simulink model "MIXER"  (R2017a)
settings: Solver=VariableStepAuto  StartTime=0.0  StopTime=50.0  RelTol=1e-3
values from neighbouring files (symbols this model uses):
  a = 1.8    [Integral.m]    (also in Koshi.m = 0; MNK.m = -5; Spline_1_0.m = -5; Spline_2_1.m = -5)
  c1 = 1    [data_mixer.m]    (also in data_mixer_for_gui.m)
  c2 = 2    [data_mixer.m]    (also in data_mixer_for_gui.m; my.m = 0.4)
  cz = 1.25    [data_mixer.m]
  F1z = uz(1)    [data_mixer.m]    (also in data_mixer_for_gui.m)
  F2z = uz(2)    [data_mixer.m]    (also in data_mixer_for_gui.m)
  Fz = 0.02    [data_mixer.m]
  k = k + 1    (= 2)    [complex_ikf.m]    (also in data_mixer.m = 0.02; data_mixer_for_gui.m = 0.02; my.m = 5)
  k1 = -10    [data_mixer.m]
  k2 = -10    [data_mixer.m]
  S = @(k)(((b1-a).^(k+1-betta))-((b1-b).^(k+1-betta)))./(k+1-betta)    [Gauss.m]    (also in Integral.m = @(k)((1/2).^(k+2/5))./(k+2/5); Nuton_Kotes.m; data_mixer.m = 1; data_mixer_for_gui.m = 1)
  X_ini = [1.5 0.5].'    [data_mixer.m]
undefined symbols (not defined in the file or in its folder): F_for_MIXER
settings Model: Creator=User  LastModifiedBy=User

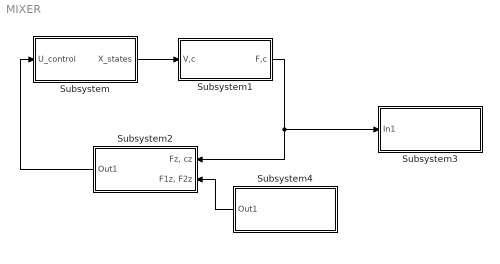
== system MIXER ==
  Subsystem : Subsystem
      mask Display:
      | color('blue');
      | disp('MIXER');
  Subsystem1 : Subsystem
      mask Display:
      | color('red');
      | disp('MEARSUREMENTS');
  Subsystem2 : Subsystem
      mask Display:
      | color('blue');
      | disp('CONTROL');
  Subsystem3 : Subsystem
      mask Display:
      | color('blue');
      | disp('DISPLAY');
  Subsystem4 : Subsystem
      mask Display:
      | color('blue');
      | disp('COMMAND\nSIGNAL');
  wires:
  Subsystem/1(X_states) -> Subsystem1/1(V,c)
  Subsystem1/1(F,c) -> Subsystem3/1(In1), Subsystem2/1("Fz, cz")
  Subsystem2/1(Out1) -> Subsystem/1(U_control)
  Subsystem4/1(Out1) -> Subsystem2/2("F1z, F2z")

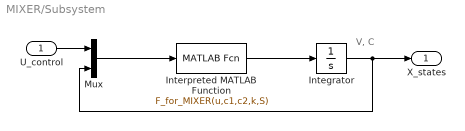
== system MIXER/Subsystem ==
  note: V, C
  U_control : Inport
  Integrator : Integrator  InitialCondition=X_ini
  Interpreted MATLAB Function : MATLABFcn  MATLABFcn=F_for_MIXER(u,c1,c2,k,S)
  Mux : Mux  Inputs=2
  X_states : Outport
  wires:
  Interpreted MATLAB Function/1 -> Integrator/1
  Integrator/1 -> Mux/2, X_states/1
  U_control/1 -> Mux/1
  Mux/1 -> Interpreted MATLAB Function/1

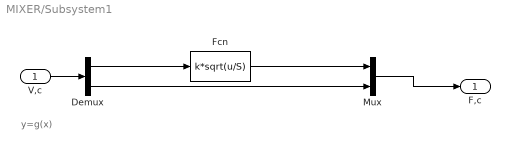
== system MIXER/Subsystem1 ==
  note: y=g(x)
  V,c : Inport
  Demux : Demux  Outputs=2
  Fcn : Fcn  Expr=k*sqrt(u/S)
  Mux : Mux  Inputs=2
  F,c : Outport
  wires:
  V,c/1 -> Demux/1
  Mux/1 -> F,c/1
  Demux/2 -> Mux/2
  Fcn/1 -> Mux/1
  Demux/1 -> Fcn/1

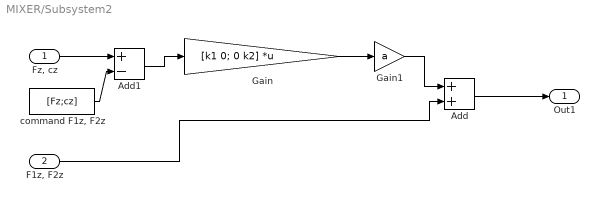
== system MIXER/Subsystem2 ==
  "Fz, cz" : Inport
  "F1z, F2z" : Inport  Port=2
  Add : Sum
  Add1 : Sum  Inputs=+-
  Gain : Gain  Gain=[k1 0; 0 k2]  Multiplication=Matrix(K*u)
  Gain1 : Gain  Gain=a
  "command F1z, F2z" : Constant  Value=[Fz;cz]
  Out1 : Outport
  wires:
  Add/1 -> Out1/1
  "F1z, F2z"/1 -> Add/2
  "command F1z, F2z"/1 -> Add1/2
  "Fz, cz"/1 -> Add1/1
  Add1/1 -> Gain/1
  Gain/1 -> Gain1/1
  Gain1/1 -> Add/1

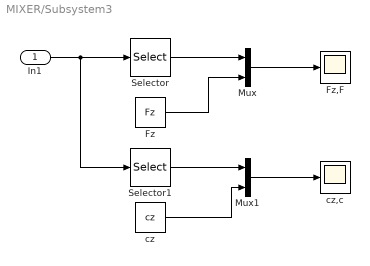
== system MIXER/Subsystem3 ==
  In1 : Inport
  Fz : Constant  Value=Fz
  Fz,F : Scope
  Mux : Mux  Inputs=2
  Mux1 : Mux  Inputs=2
  Selector : Selector  InputPortWidth=2  IndexOptions=Index vector (dialog)  Indices=1  OutputSizes=1
  Selector1 : Selector  InputPortWidth=2  IndexOptions=Index vector (dialog)  Indices=2  OutputSizes=1
  cz : Constant  Value=cz
  cz,c : Scope
  wires:
  Selector/1 -> Mux/1
  Fz/1 -> Mux/2
  In1/1 -> Selector1/1, Selector/1
  Selector1/1 -> Mux1/1
  cz/1 -> Mux1/2
  Mux/1 -> Fz,F/1
  Mux1/1 -> cz,c/1

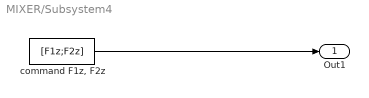
== system MIXER/Subsystem4 ==
  "command F1z, F2z" : Constant  Value=[F1z;F2z]
  Out1 : Outport
  wires:
  "command F1z, F2z"/1 -> Out1/1
